simulink model "testLQR"  (R2017b)
settings: Solver=VariableStepAuto  StartTime=0.0  StopTime=20  RelTol=1e-3
values from neighbouring files (symbols this model uses):
  Ax = [zeros(2), eye(2), zeros(2,1) ... (first row only)    [ComputeLQR.m]
  Bx = [0;0;0;0;2]    [ComputeLQR.m]    (also in RobotDynamics.m = [tx;Rb*tx])
  K = Kx    [ComputeLQR.m]
settings Model: Creator=qrx  LastModifiedBy=qrx

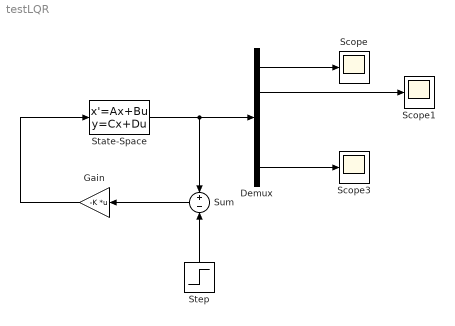
== system testLQR ==
  Demux : Demux  Outputs=5
  Gain : Gain  Gain=-K  Multiplication=Matrix(K*u)
  Scope : Scope
  Scope1 : Scope
  Scope3 : Scope
  State-Space : StateSpace  A=Ax  B=Bx  C=eye(5)  D=zeros(5,1)  InitialCondition=0
  Step : Step  Time=0  Before=[0 0 0 0 0]  After=[50 0 0 0 0]  SampleTime=0
  Sum : Sum  Inputs=+-
  wires:
  Gain/1 -> State-Space/1
  Sum/1 -> Gain/1
  State-Space/1 -> Sum/1, Demux/1
  Step/1 -> Sum/2
  Demux/1 -> Scope/1
  Demux/2 -> Scope1/1
  Demux/5 -> Scope3/1
